simulink model "L5Ex1"  (R2020b)
settings: Solver=VariableStepAuto  StartTime=0.0  StopTime=10.0  RelTol=1e-3
undefined symbols (not defined in the file): magnitude
libraries: powerlib x3
settings Model: Creator=Vedant Nath  LastModifiedBy=Vedant Nath

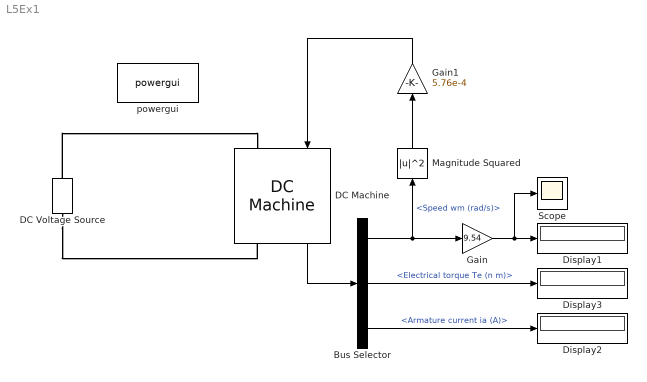
== system L5Ex1 ==
  Bus Selector : BusSelector  OutputSignals=Speed wm (rad/s),Electrical torque Te (n m),Armature current ia (A)
  DC Machine : powerlib/Machines/DC Machine  PresetModel=No  MechanicalLoad=Torque TL  FieldType=Permanent magnet  ShowDetailedParameters=on  MeasurementBus=off  RLa="[ 2  0.011]"  RLf="[ 240  120]"  Laf=1.8  MachineConstant=Torque constant (N.m/A)  Ke=1.8  Kt=1.26  J=0.05  Bm=0  Tf=0  w0=1  Ifinit=1  TsPowergui=0  TsBlock=-1
  DC Voltage Source : powerlib/Electrical Sources/DC Voltage Source  Amplitude=105  Measurements=None
  Display1 : Display
  Display2 : Display
  Display3 : Display
  Gain : Gain  Gain=9.54
  Gain1 : Gain  Gain=5.76e-4
  Magnitude Squared : Math  Operator=magnitude^2  SaturateOnIntegerOverflow=on
  Scope : Scope
  powergui : powerlib/powergui  Priority=1  SimulationMode=Continuous  SampleTime=50e-6  frequency=60  Iterations=50  frequencyindice=0  Pbase=100e6  ErrMax=1e-4  UnitsV=kV  UnitsW=MW  buscounter=0  FunctionMessages=off  echomessages=off  EnableUseOfTLC=off  CurrentSourceSwitches=off  DisableSnubberDevices=off  DisableRonSwitches=off  DisableVfSwitches=off  DisplayEquations=off  AutomaticDiscreteSolvers=off  SolverType=Tustin/Backward Euler (TBE)  Interpol=off  ExternalGateDelay=off  methode=off  Ts=100  x0status=zero  SPID=on  SwTol=0  HookPort=off  NonlinearTolerance=1e-4  nMaxIteration=100  ContinueOnMaxIteration=off  RestoreLinks=warning  ResistiveCurrentMeasurement=off  Frange=[0:2:500]  Ylog=off  Xlog=on  ShowGrid=off  save=off  variable=ZData  structure=0  ZoomFFT=off  StartTime=0.0  cycles=1  DisplayStyle=1  fundamental=60  FreqAxis=off  MaxFrequency=1000  frequencyindicesteady=1  RmsSteady=1  display=off
  wires:
  Gain/1 -> Display1/1, Scope/1
  DC Machine/1 -> Bus Selector/1
  Gain1/1 -> DC Machine/1
  Bus Selector/3 -> Display2/1  "<Armature current ia (A)>"
  Bus Selector/2 -> Display3/1  "<Electrical torque Te (n m)>"
  Bus Selector/1 -> Magnitude Squared/1, Gain/1  "<Speed wm (rad/s)>"
  Magnitude Squared/1 -> Gain1/1
  connections:
  DC Voltage Source/LConn1 -- DC Machine/RConn1
  DC Voltage Source/RConn1 -- DC Machine/LConn1
